simulink model "Q2_sim"  (R2022b)
settings: Solver=VariableStepAuto  StartTime=0.0  StopTime=100  RelTol=1e-3
settings Model: Creator=beni  LastModifiedBy=beni

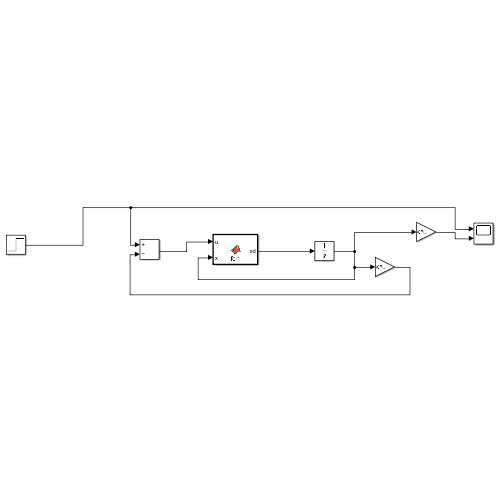
[thumbnail: Simulink's stored preview of the top-level diagram]
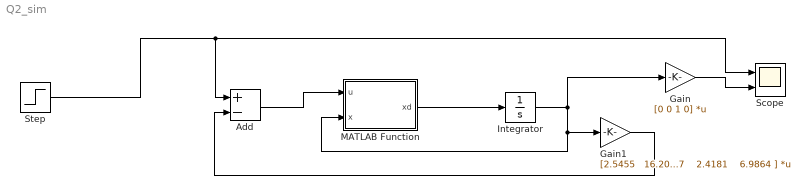
== system Q2_sim ==
  Add : Sum  Inputs=+-
  Gain : Gain  Gain=[0 0 1 0]  Multiplication=Matrix(K*u)
  Gain1 : Gain  Gain=|  Multiplication=Matrix(K*u)
      | [2.5455   16.2067    2.4181    6.9864
      | ]
  Integrator : Integrator  InitialCondition=[0;0;0;0]
  MATLAB Function : MATLAB Function  TreatAsAtomicUnit=on
  Scope : Scope  NumInputPorts=2
  Step : Step  SampleTime=0
  wires:
  MATLAB Function/1(xd) -> Integrator/1
  Integrator/1 -> MATLAB Function/2(x), Gain1/1, Gain/1
  Gain/1 -> Scope/2
  Add/1 -> MATLAB Function/1(u)
  Gain1/1 -> Add/2
  Step/1 -> Add/1, Scope/1

== matlab function Q2_sim/MATLAB Function ==
  data: u input; xd output; x input
function xd= fcn(u,x)

A1 =[0    1.0000         0         0;
   -1.7560   -0.0591    0.0109    0.0005;
         0         0         0    1.0000;
    0.0139    0.0005   -1.3810   -0.0595];

B1=[0;
  -16.0100;
         0;
   38.8400];

xd = A1*x+B1*u;
